simulink model "EC_Motor"  (R2023a)
settings: Solver=VariableStepAuto  StartTime=0.0  StopTime=simtime  FixedStep=0.01  MaxStep=0.001  RelTol=1e-3
undefined symbols (not defined in the file): J_Mo, k, k_M, L, M_L, phi_R, phi_St, Q, R, u_M_fin, u_M_ini
settings Model: Creator=fycce  LastModifiedBy=fycce
settings DataIOCC: SaveOutput=off  SaveTime=off  ReturnWorkspaceOutputs=off

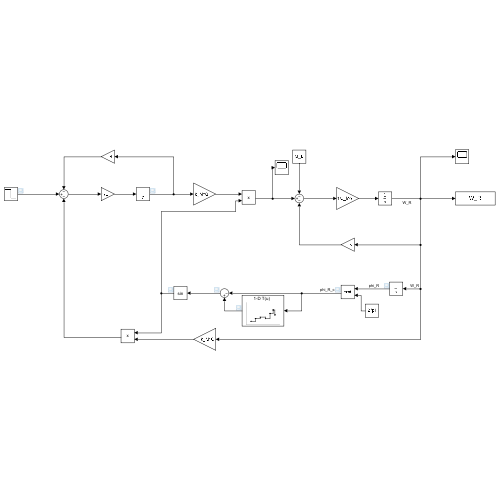
[thumbnail: Simulink's stored preview of the top-level diagram]
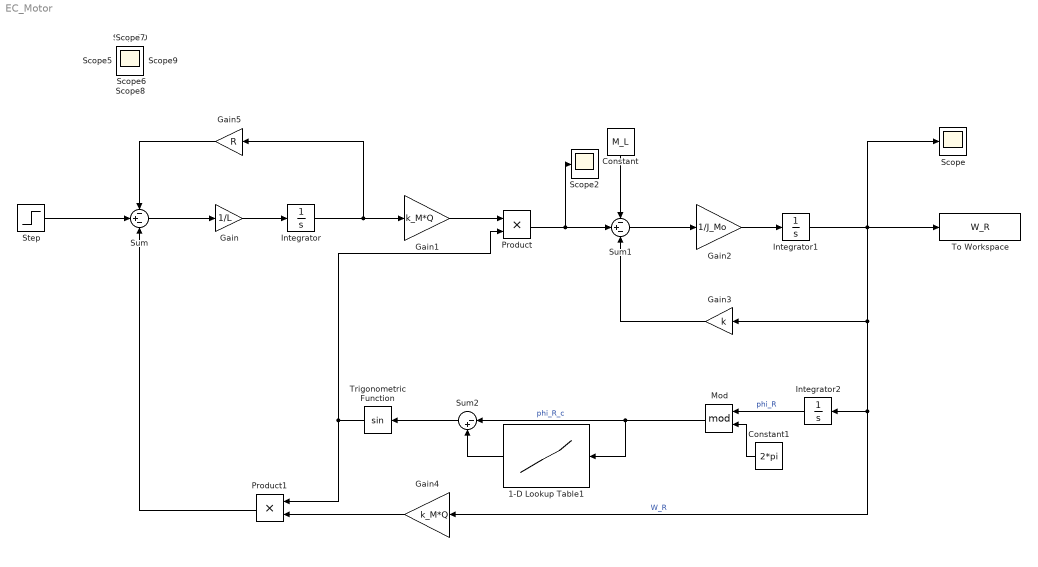
== system EC_Motor ==
  1-D Lookup Table1 : Lookup_n-D  NumberOfTableDimensions=1  BreakpointsForDimension1=phi_R  Table=phi_St  InterpMethod=Flat  InternalRulePriority=Speed  RndMeth=Simplest
  Constant : Constant  Value=M_L
  Constant1 : Constant  Value=2*pi
  Gain : Gain  Gain=1/L
  Gain1 : Gain  Gain=k_M*Q
  Gain2 : Gain  Gain=1/J_Mo
  Gain3 : Gain  Gain=k
  Gain4 : Gain  Gain=k_M*Q
  Gain5 : Gain  Gain=R
  Integrator : Integrator
  Integrator1 : Integrator
  Integrator2 : Integrator
  Mod : Math  Operator=mod
  Product : Product
  Product1 : Product
  Scope{,1..10} (11 alike) : Scope
  Step : Step  Time=0.25  Before=u_M_ini  After=u_M_fin  SampleTime=0
  Sum : Sum  Inputs=-+-
  Sum1 : Sum  Inputs=-+-
  Sum2 : Sum  Inputs=|-+
  To Workspace : ToWorkspace  VariableName=W_R  SaveFormat=Timeseries  SampleTime=-1
  Trigonometric Function : Trigonometry
  wires:
  Step/1 -> Sum/2
  Sum/1 -> Gain/1
  Gain/1 -> Integrator/1
  Integrator/1 -> Gain5/1, Gain1/1
  Gain1/1 -> Product/1
  Product/1 -> Scope2/1, Sum1/2
  Constant/1 -> Sum1/1
  Sum1/1 -> Gain2/1
  Gain2/1 -> Integrator1/1
  Integrator1/1 -> Gain4/1, Integrator2/1, Gain3/1, Scope/1, To Workspace/1  "W_R"
  Gain3/1 -> Sum1/3
  Integrator2/1 -> Mod/1  "phi_R"
  Sum2/1 -> Trigonometric Function/1
  Trigonometric Function/1 -> Product1/1, Product/2
  Gain4/1 -> Product1/2
  Product1/1 -> Sum/3
  Gain5/1 -> Sum/1
  1-D Lookup Table1/1 -> Sum2/2
  Mod/1 -> 1-D Lookup Table1/1, Sum2/1  "phi_R_c"
  Constant1/1 -> Mod/2
